simulink model "Second_Order_Sytsem_PD_Controller_Series_Parellel_Ideal"  (R2024b)
settings: Solver=VariableStepAuto  StartTime=0.0  StopTime=10.0  RelTol=1e-3
settings Model: Creator=Ahmad  LastModifiedBy=Ahmad

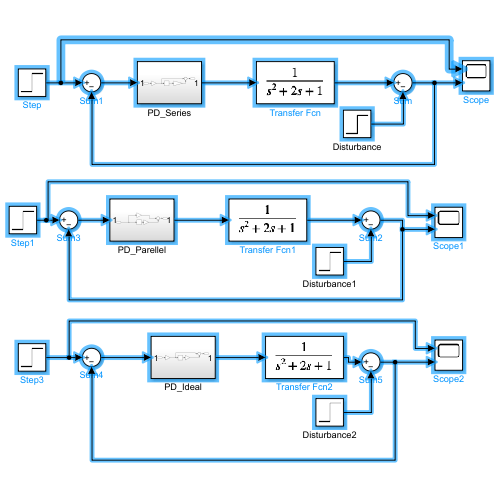
[thumbnail: Simulink's stored preview of the top-level diagram]
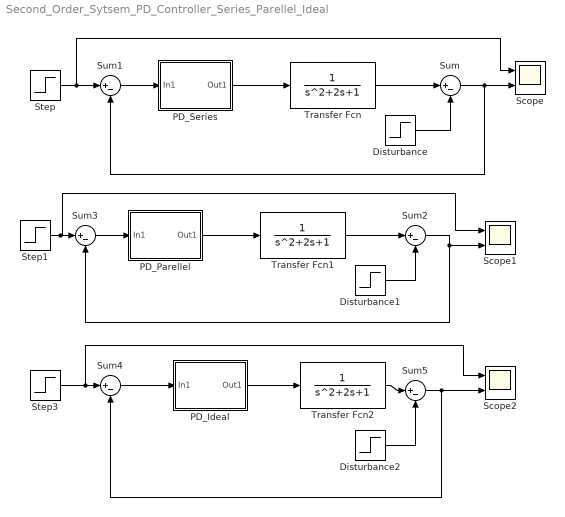
== system Second_Order_Sytsem_PD_Controller_Series_Parellel_Ideal ==
  Disturbance : Step  After=0.5  SampleTime=0
  Disturbance1 : Step  After=0.5  SampleTime=0
  Disturbance2 : Step  After=0.5  SampleTime=0
  PD_Ideal : Subsystem
  PD_Parellel : Subsystem
  PD_Series : Subsystem
  Scope : Scope  NumInputPorts=2
  Scope1 : Scope  NumInputPorts=2
  Scope2 : Scope  NumInputPorts=2
  Step : Step  SampleTime=0
  Step1 : Step  SampleTime=0
  Step3 : Step  SampleTime=0
  Sum{,1..5} (6 alike) : Sum  Inputs=|+-
  Transfer Fcn : TransferFcn
  Transfer Fcn1 : TransferFcn
  Transfer Fcn2 : TransferFcn
  wires:
  Sum5/1 -> Sum4/2, Scope2/2
  PD_Parellel/1(Out1) -> Transfer Fcn1/1
  Transfer Fcn2/1 -> Sum5/1
  Sum3/1 -> PD_Parellel/1(In1)
  Step1/1 -> Scope1/1, Sum3/1
  Sum2/1 -> Scope1/2, Sum3/2
  Sum/1 -> Sum1/2, Scope/2
  Disturbance/1 -> Sum/2
  Step3/1 -> Sum4/1, Scope2/1
  Disturbance2/1 -> Sum5/2
  Sum1/1 -> PD_Series/1(In1)
  Disturbance1/1 -> Sum2/2
  PD_Series/1(Out1) -> Transfer Fcn/1
  Step/1 -> Scope/1, Sum1/1
  Transfer Fcn/1 -> Sum/1
  Transfer Fcn1/1 -> Sum2/1
  PD_Ideal/1(Out1) -> Transfer Fcn2/1
  Sum4/1 -> PD_Ideal/1(In1)

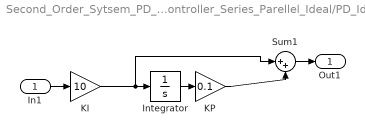
== system Second_Order_Sytsem_PD_Controller_Series_Parellel_Ideal/PD_Ideal ==
  In1 : Inport
  Integrator : Integrator
  KI : Gain  Gain=10
  KP : Gain  Gain=0.1
  Sum1 : Sum  Inputs=|++
  Out1 : Outport
  wires:
  KI/1 -> Integrator/1, Sum1/1
  Integrator/1 -> KP/1
  In1/1 -> KI/1
  KP/1 -> Sum1/2
  Sum1/1 -> Out1/1

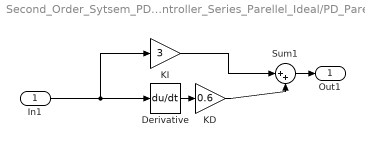
== system Second_Order_Sytsem_PD_Controller_Series_Parellel_Ideal/PD_Parellel ==
  In1 : Inport
  Derivative : Derivative
  KD : Gain  Gain=0.6
  KI : Gain  Gain=3
  Sum1 : Sum  Inputs=|++
  Out1 : Outport
  wires:
  In1/1 -> Derivative/1, KI/1
  Derivative/1 -> KD/1
  KD/1 -> Sum1/2
  Sum1/1 -> Out1/1
  KI/1 -> Sum1/1

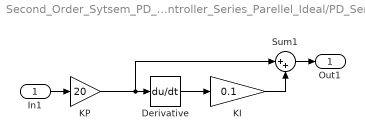
== system Second_Order_Sytsem_PD_Controller_Series_Parellel_Ideal/PD_Series ==
  In1 : Inport
  Derivative : Derivative
  KI : Gain  Gain=0.1
  KP : Gain  Gain=20
  Sum1 : Sum  Inputs=|++
  Out1 : Outport
  wires:
  KP/1 -> Derivative/1, Sum1/1
  Derivative/1 -> KI/1
  In1/1 -> KP/1
  KI/1 -> Sum1/2
  Sum1/1 -> Out1/1
